simulink model "Tagekilometerzaehler"  (R2017a)
settings: Solver=ode1  StartTime=0.0  StopTime=1  FixedStep=0.001  RelTol=1e-3
PostLoadFcn:
  | , if any(exist('dsrtsu_mdlpostloadfcn', 'file') == [2, 3, 6]), try dsrtsu_mdlpostloadfcn('Execute', bdroot); catch fprintf('Error in PostLoadFcn (dsrtsu_mdlpostloadfcn) for model "%s":\n %s\n', bdroot, lasterr); end, end,
undefined symbols (not defined in the file): DiscIntNeverNeededParam
libraries: simulink x2
Description:
  | Standard RTI1401 template.
  | Supported Matlab version:  R2017a.
settings Model: Tag=RTI1401  DSRTSU_INTERNAL_RTI_VER=500  DSRTSU_INTERNAL_RTI_TYPE=rti1401  Creator=DeltaRacing  LastModifiedBy=DeltaRacing
settings OptimizationCC: BlockReduction=off  OptimizeBlockIOStorage=off  BufferReuse=off  GlobalBufferReuse=off  ExpressionFolding=off  LocalBlockOutputs=off
settings HardwareCC: ProdBitPerPointer=32  ProdBitPerSizeT=32  ProdBitPerPtrDiffT=32  ProdLargestAtomicInteger=Integer  ProdEndianess=BigEndian  ProdWordSize=32  ProdHWDeviceType=Custom Processor->Custom  TargetIntDivRoundTo=Zero  TargetEndianess=BigEndian  TargetHWDeviceType=Custom Processor->Custom
settings SFSimCC: MATLABDynamicMemAlloc=off
settings RTWCC: SystemTargetFile=rti1401.tlc  MakeCommand=make_rti  TemplateMakefile=rti1401.tmf  Description=dSPACE DS1401 Hardware Platform
settings STFCustomTargetCC: ParMdlRefBuildCompliant=on  MatFileLogging=on  GRTInterface=off  SystemTargetFile=rti1401.tlc
settings GRTTargetCC: TargetLangStandard=C89/C90 (ANSI)  CompOptLevelCompliant=off  ConcurrentExecutionCompliant=off  CombineOutputUpdateFcns=off  CPPClassGenCompliant=off  UseToolchainInfoCompliant=off
settings ConfigComp: CovMetricSettings=dswe

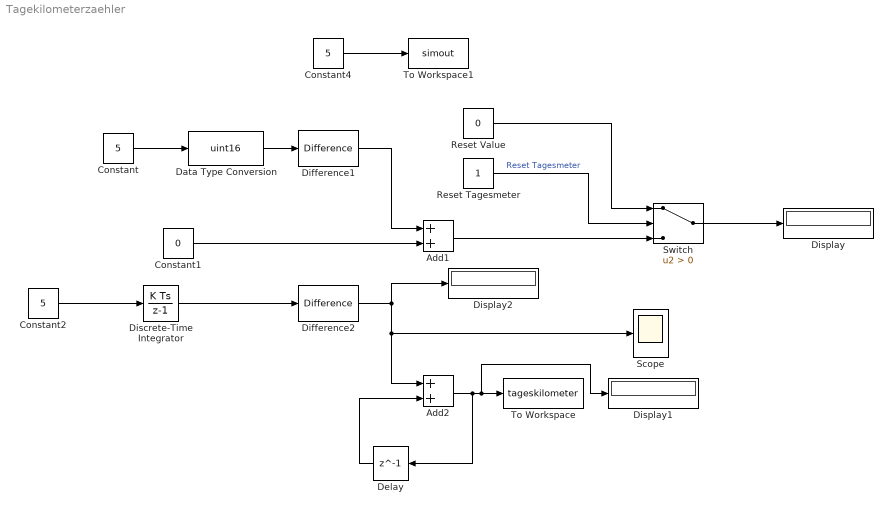
== system Tagekilometerzaehler ==
  Add1 : Sum
  Add2 : Sum
  Constant : Constant  Value=5
  Constant1 : Constant  Value=0
  Constant2 : Constant  Value=5
  Constant4 : Constant  Value=5
  Data Type Conversion : DataTypeConversion  OutDataTypeStr=uint16
  Delay : Delay  DelayLength=1
  Difference1 : simulink/Discrete/Difference  ICPrevInput=0.0  OutMin=[]  OutMax=[]  OutDataType=fixdt(1, 16)  OutScaling=2^-10  DoSatur=off
  Difference2 : simulink/Discrete/Difference  ICPrevInput=0.0  OutMin=[]  OutMax=[]  OutDataType=fixdt(1, 16)  OutScaling=2^-10  DoSatur=off
  Discrete-Time Integrator : DiscreteIntegrator  InitialConditionSetting=State (most efficient)  SampleTime=-1  ICPrevOutput=DiscIntNeverNeededParam  ICPrevScaledInput=DiscIntNeverNeededParam
  Display : Display
  Display1 : Display
  Display2 : Display
  Reset Tagesmeter : Constant
  Reset Value : Constant  Value=0  OutDataTypeStr=uint16
  Scope : Scope
  Switch : Switch  Criteria=u2 > Threshold
  To Workspace : ToWorkspace  VariableName=tageskilometer  SaveFormat=Timeseries  SampleTime=-1
  To Workspace1 : ToWorkspace  VariableName=simout  SaveFormat=Timeseries  SampleTime=-1
  wires:
  Constant1/1 -> Add1/2
  Difference1/1 -> Add1/1
  Data Type Conversion/1 -> Difference1/1
  Switch/1 -> Display/1
  Add1/1 -> Switch/3
  Reset Value/1 -> Switch/1
  Reset Tagesmeter/1 -> Switch/2  "Reset Tagesmeter"
  Constant/1 -> Data Type Conversion/1
  Delay/1 -> Add2/2
  Discrete-Time Integrator/1 -> Difference2/1
  Difference2/1 -> Display2/1, Scope/1, Add2/1
  Add2/1 -> Delay/1, Display1/1, To Workspace/1
  Constant2/1 -> Discrete-Time Integrator/1
  Constant4/1 -> To Workspace1/1
